simulink model "dllModel"  (R2015b)
settings: Solver=FixedStepDiscrete  StartTime=0.0  StopTime=10  FixedStep=0.1  RelTol=1e-3
values from neighbouring files (symbols this model uses):
  K = Simulink.Parameter    [dllModel_init.m]
  K2 = Simulink.Parameter    [dllModel_init.m]
settings Model: SimulationMode=accelerator  Creator=C3038028  LastModifiedBy=C3038028
settings DataIOCC: LimitDataPoints=off  SaveOutput=off  SignalLogging=off  VisualizeSimOutput=off  SaveTime=off
settings OptimizationCC: BlockReduction=off  ConditionallyExecuteInputs=off  DefaultParameterBehavior=Inlined  DefaultUnderspecifiedDataType=single  OptimizeModelRefInitCode=on  LifeSpan=Inf
settings HardwareCC: TargetBitPerPointer=64  TargetLongLongMode=on  TargetIntDivRoundTo=Zero  TargetEndianess=LittleEndian  TargetWordSize=64  TargetHWDeviceType=MATLAB Host  ProdEqTarget=off
settings RTWCC: SystemTargetFile=ert_shrlib.tlc  TemplateMakefile=ert_default_tmf  Description=Embedded Coder (host-based shared library target)  Toolchain=Microsoft Windows SDK v7.1 | nmake (64-bit Windows)
settings CodeAppCC: IgnoreCustomStorageClasses=off
settings STFCustomTargetCC: GenerateSampleERTMain=on  ParMdlRefBuildCompliant=on  CompOptLevelCompliant=on  ConcurrentExecutionCompliant=off  GeneratePreprocessorConditionals=Use local settings  CombineOutputUpdateFcns=on  ERTCustomFileBanners=on  SupportContinuousTime=off  SupportNonInlinedSFcns=off  MATLABClassNameForMDSCustomization=Simulink.SoftwareTarget.ERTCustomization  ModelStepFunctionPrototypeControlCompliant=on  CPPClassGenCompliant=off  GRTInterface=off  UseToolchainInfoCompliant=on  SystemTargetFile=ert_shrlib.tlc
settings ERTTargetCC: GenerateSampleERTMain=on  ConcurrentExecutionCompliant=off  ERTFirstTimeCompliant=off  CPPClassGenCompliant=off  InlinedParameterPlacement=NonHierarchical  ERTCustomFileTemplate=example_file_process.tlc

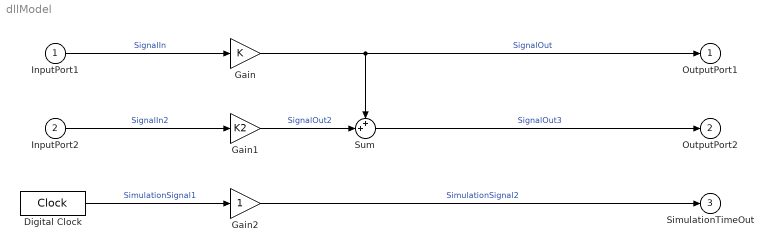
== system dllModel ==
  InputPort1 : Inport  OutDataTypeStr=single
  InputPort2 : Inport  Port=2  OutDataTypeStr=uint16
  Digital Clock : DigitalClock  SampleTime=0.1
  Gain : Gain  Gain=K  OutDataTypeStr=single
  Gain1 : Gain  Gain=K2  OutDataTypeStr=uint16
  Gain2 : Gain  OutDataTypeStr=Inherit: Same as input
  Sum : Sum  Inputs=++|
  OutputPort1 : Outport
  OutputPort2 : Outport  Port=2
  SimulationTimeOut : Outport  Port=3
  wires:
  InputPort1/1 -> Gain/1  "SignalIn"
  Gain/1 -> OutputPort1/1, Sum/1  "SignalOut"
  InputPort2/1 -> Gain1/1  "SignalIn2"
  Sum/1 -> OutputPort2/1  "SignalOut3"
  Gain1/1 -> Sum/2  "SignalOut2"
  Digital Clock/1 -> Gain2/1  "SimulationSignal1"
  Gain2/1 -> SimulationTimeOut/1  "SimulationSignal2"
